simulink model "NB_simulink"  (R2023a)
settings: Solver=VariableStepAuto  StartTime=0.0  StopTime=974  RelTol=1e-3
undefined symbols (not defined in the file): g_i, g_p
libraries: simulink x6
settings Model: Creator=usradmin  LastModifiedBy=usradmin

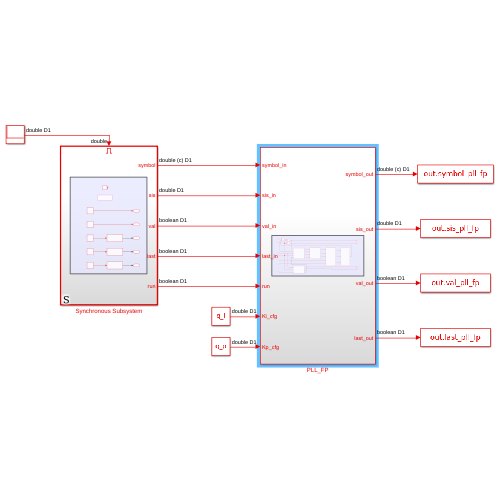
[thumbnail: Simulink's stored preview of the top-level diagram]
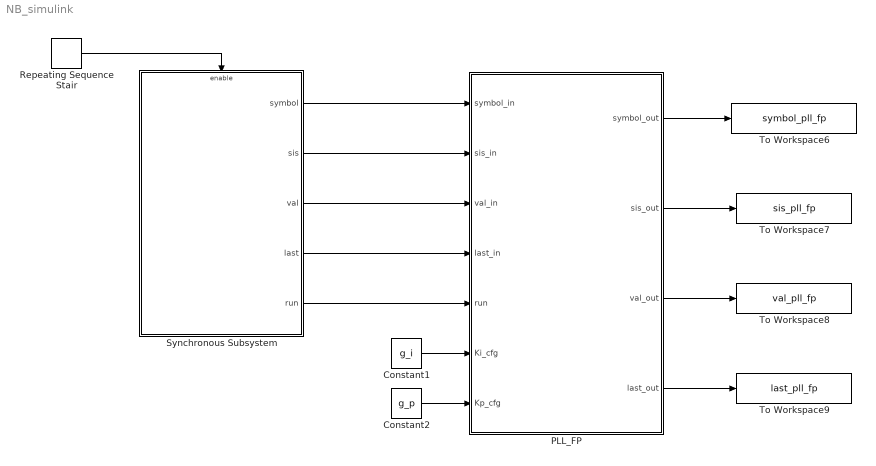
== system NB_simulink ==
  Constant1 : Constant  Value=g_i  SampleTime=-1
  Constant2 : Constant  Value=g_p  SampleTime=-1
  PLL_FP : Subsystem
  Repeating Sequence Stair : simulink/Sources/Repeating Sequence Stair  OutValues=1  tsamp=1  OutMin=[]  OutMax=[]  OutDataTypeStr=double  OutputDataTypeScalingMode=double  OutDataType=fixdt(0,8)  ConRadixGroup=Best Precision: Vector-wise  OutScaling=2^-12
  Synchronous Subsystem : Subsystem
  To Workspace6 : ToWorkspace  VariableName=symbol_pll_fp  SampleTime=-1
      settings: Save2DSignal=2-D array (concatenate along first dimension)
  To Workspace7 : ToWorkspace  VariableName=sis_pll_fp  SampleTime=-1
      settings: Save2DSignal=2-D array (concatenate along first dimension)
  To Workspace8 : ToWorkspace  VariableName=val_pll_fp  SampleTime=-1
      settings: Save2DSignal=2-D array (concatenate along first dimension)
  To Workspace9 : ToWorkspace  VariableName=last_pll_fp  SampleTime=-1
      settings: Save2DSignal=2-D array (concatenate along first dimension)
  wires:
  Repeating Sequence Stair/1 -> Synchronous Subsystem/Enable
  Synchronous Subsystem/1(symbol) -> PLL_FP/1(symbol_in)
  PLL_FP/1(symbol_out) -> To Workspace6/1
  Synchronous Subsystem/4(last) -> PLL_FP/4(last_in)
  PLL_FP/3(val_out) -> To Workspace8/1
  PLL_FP/4(last_out) -> To Workspace9/1
  Constant1/1 -> PLL_FP/6(Ki_cfg)
  Constant2/1 -> PLL_FP/7(Kp_cfg)
  Synchronous Subsystem/2(sis) -> PLL_FP/2(sis_in)
  Synchronous Subsystem/5(run) -> PLL_FP/5(run)
  Synchronous Subsystem/3(val) -> PLL_FP/3(val_in)
  PLL_FP/2(sis_out) -> To Workspace7/1

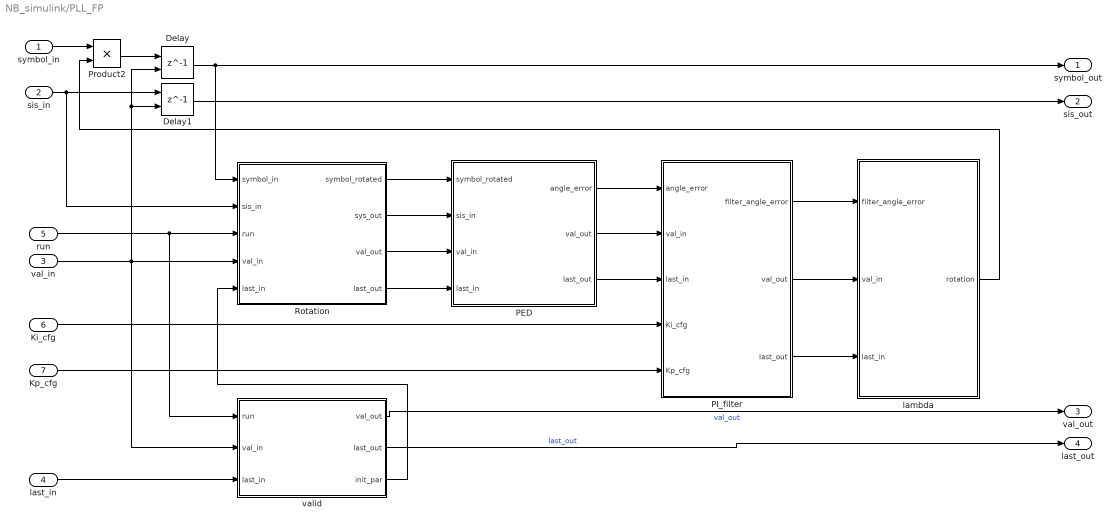
== system NB_simulink/PLL_FP ==
  symbol_in : Inport
  sis_in : Inport  Port=2
  val_in : Inport  Port=3
  last_in : Inport  Port=4
  run : Inport  Port=5
  Ki_cfg : Inport  Port=6
  Kp_cfg : Inport  Port=7
  Delay : Delay  DelayLength=1  InitialCondition=0  ShowEnablePort=on
      settings: InputPortMap=u0,e6
  Delay1 : Delay  DelayLength=1  InitialCondition=0  ShowEnablePort=on
      settings: InputPortMap=u0,e6
  PED : Subsystem
  PI_filter : Subsystem
  Product2 : Product
  Rotation : Subsystem
  lambda : Subsystem
  valid : MATLAB Function  TreatAsAtomicUnit=on
  symbol_out : Outport
  sis_out : Outport  Port=2
  val_out : Outport  Port=3
  last_out : Outport  Port=4
  wires:
  lambda/1(rotation) -> Product2/2
  PED/1(angle_error) -> PI_filter/1(angle_error)
  PI_filter/1(filter_angle_error) -> lambda/1(filter_angle_error)
  Rotation/1(symbol_rotated) -> PED/1(symbol_rotated)
  Product2/1 -> Delay/1
  symbol_in/1 -> Product2/1
  sis_in/1 -> Delay1/1, Rotation/2(sis_in)
  Rotation/2(sys_out) -> PED/2(sis_in)
  val_in/1 -> Delay1/2, Delay/2, valid/2(val_in), Rotation/4(val_in)
  last_in/1 -> valid/3(last_in)
  Rotation/3(val_out) -> PED/3(val_in)
  Rotation/4(last_out) -> PED/4(last_in)
  PED/2(val_out) -> PI_filter/2(val_in)
  PED/3(last_out) -> PI_filter/3(last_in)
  PI_filter/2(val_out) -> lambda/2(val_in)
  PI_filter/3(last_out) -> lambda/3(last_in)
  Delay/1 -> Rotation/1(symbol_in), symbol_out/1
  valid/1(val_out) -> val_out/1  "val_out"
  valid/2(last_out) -> last_out/1  "last_out"
  Ki_cfg/1 -> PI_filter/4(Ki_cfg)
  Kp_cfg/1 -> PI_filter/5(Kp_cfg)
  run/1 -> valid/1(run), Rotation/3(run)
  Delay1/1 -> sis_out/1
  valid/3(init_par) -> Rotation/5(last_in)

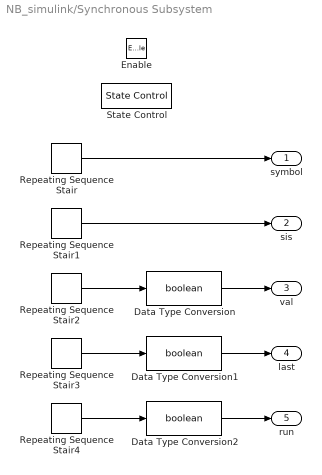
== system NB_simulink/Synchronous Subsystem ==
  Enable : EnablePort  ShowOutputPort=on
  Data Type Conversion : DataTypeConversion  OutDataTypeStr=boolean  SaturateOnIntegerOverflow=off  RndMeth=Floor
  Data Type Conversion1 : DataTypeConversion  OutDataTypeStr=boolean  SaturateOnIntegerOverflow=off  RndMeth=Floor
  Data Type Conversion2 : DataTypeConversion  OutDataTypeStr=boolean  SaturateOnIntegerOverflow=off  RndMeth=Floor
  Repeating Sequence Stair : simulink/Sources/Repeating Sequence Stair  OutValues=symbol_cc  tsamp=1  OutMin=[]  OutMax=[]  OutDataTypeStr=double  OutputDataTypeScalingMode=double  OutDataType=fixdt(0,8)  ConRadixGroup=Best Precision: Vector-wise  OutScaling=2^-12
  Repeating Sequence Stair1 : simulink/Sources/Repeating Sequence Stair  OutValues=sis_cc  tsamp=1  OutMin=[]  OutMax=[]  OutDataTypeStr=double  OutputDataTypeScalingMode=double  OutDataType=fixdt(0,8)  ConRadixGroup=Best Precision: Vector-wise  OutScaling=2^-12
  Repeating Sequence Stair2 : simulink/Sources/Repeating Sequence Stair  OutValues=val_cc  tsamp=1  OutMin=[]  OutMax=[]  OutDataTypeStr=double  OutputDataTypeScalingMode=double  OutDataType=fixdt(0,8)  ConRadixGroup=Best Precision: Vector-wise  OutScaling=2^-12
  Repeating Sequence Stair3 : simulink/Sources/Repeating Sequence Stair  OutValues=last_cc  tsamp=1  OutMin=[]  OutMax=[]  OutDataTypeStr=double  OutputDataTypeScalingMode=double  OutDataType=fixdt(0,8)  ConRadixGroup=Best Precision: Vector-wise  OutScaling=2^-12
  Repeating Sequence Stair4 : simulink/Sources/Repeating Sequence Stair  OutValues=run_cc  tsamp=1  OutMin=[]  OutMax=[]  OutDataTypeStr=double  OutputDataTypeScalingMode=double  OutDataType=fixdt(0,8)  ConRadixGroup=Best Precision: Vector-wise  OutScaling=2^-12
  State Control : StateControl  StateControl=Synchronous
  symbol : Outport  VectorParamsAs1DForOutWhenUnconnected=off
  sis : Outport  Port=2  VectorParamsAs1DForOutWhenUnconnected=off
  val : Outport  Port=3  VectorParamsAs1DForOutWhenUnconnected=off
  last : Outport  Port=4  VectorParamsAs1DForOutWhenUnconnected=off
  run : Outport  Port=5  VectorParamsAs1DForOutWhenUnconnected=off
  wires:
  Repeating Sequence Stair/1 -> symbol/1
  Repeating Sequence Stair1/1 -> sis/1
  Repeating Sequence Stair3/1 -> Data Type Conversion1/1
  Repeating Sequence Stair2/1 -> Data Type Conversion/1
  Repeating Sequence Stair4/1 -> Data Type Conversion2/1
  Data Type Conversion/1 -> val/1
  Data Type Conversion1/1 -> last/1
  Data Type Conversion2/1 -> run/1

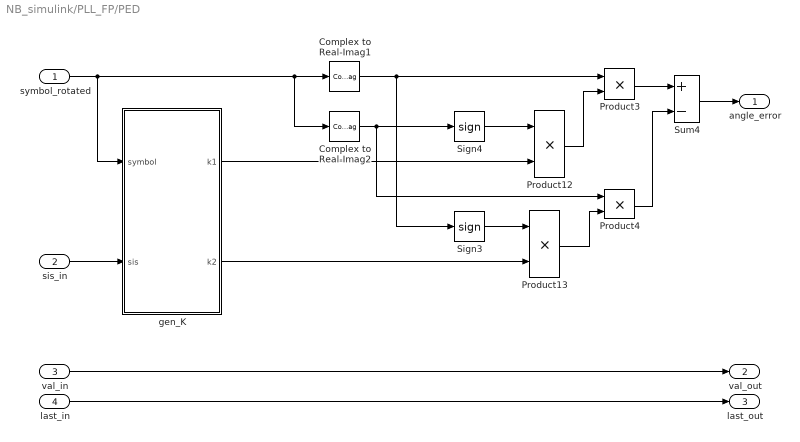
== system NB_simulink/PLL_FP/PED ==
  symbol_rotated : Inport
  sis_in : Inport  Port=2
  val_in : Inport  Port=3
  last_in : Inport  Port=4
  Complex to Real-Imag1 : ComplexToRealImag  Output=Imag
  Complex to Real-Imag2 : ComplexToRealImag  Output=Real
  Product{3..4,12..13} (4 alike) : Product
  Sign3 : Signum
  Sign4 : Signum
  Sum4 : Sum  Inputs=+-
  gen_K : MATLAB Function  TreatAsAtomicUnit=on
  angle_error : Outport
  val_out : Outport  Port=2
  last_out : Outport  Port=3
  wires:
  Product3/1 -> Sum4/1
  Product12/1 -> Product3/2
  gen_K/2(k2) -> Product13/2
  gen_K/1(k1) -> Product12/2
  Sum4/1 -> angle_error/1
  Product4/1 -> Sum4/2
  Sign3/1 -> Product13/1
  Sign4/1 -> Product12/1
  symbol_rotated/1 -> gen_K/1(symbol), Complex to Real-Imag2/1, Complex to Real-Imag1/1
  Complex to Real-Imag1/1 -> Product3/1, Sign3/1
  Complex to Real-Imag2/1 -> Sign4/1, Product4/1
  Product13/1 -> Product4/2
  sis_in/1 -> gen_K/2(sis)
  val_in/1 -> val_out/1
  last_in/1 -> last_out/1

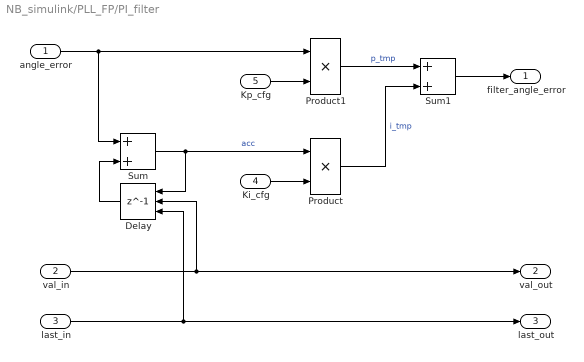
== system NB_simulink/PLL_FP/PI_filter ==
  angle_error : Inport
  val_in : Inport  Port=2
  last_in : Inport  Port=3
  Ki_cfg : Inport  Port=4
  Kp_cfg : Inport  Port=5
  Delay : Delay  DelayLength=1  ExternalReset=Level  ShowEnablePort=on
      settings: InputPortMap=u0,e6,r5
  Product : Product
  Product1 : Product
  Sum : Sum
  Sum1 : Sum
  filter_angle_error : Outport
  val_out : Outport  Port=2
  last_out : Outport  Port=3
  wires:
  Sum/1 -> Delay/1, Product/1  "acc"
  Delay/1 -> Sum/2
  Product1/1 -> Sum1/1  "p_tmp"
  Sum1/1 -> filter_angle_error/1
  angle_error/1 -> Sum/1, Product1/1
  Product/1 -> Sum1/2  "i_tmp"
  val_in/1 -> Delay/2, val_out/1
  last_in/1 -> Delay/3, last_out/1
  Ki_cfg/1 -> Product/2
  Kp_cfg/1 -> Product1/2

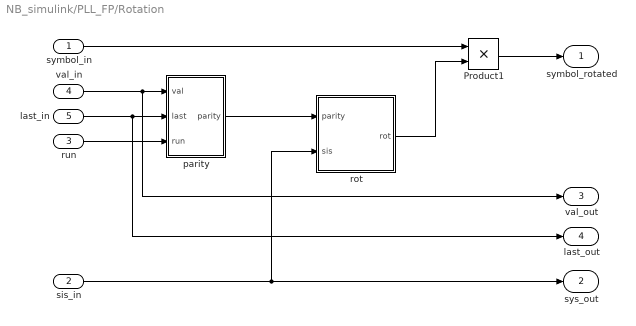
== system NB_simulink/PLL_FP/Rotation ==
  symbol_in : Inport
  sis_in : Inport  Port=2
  run : Inport  Port=3
  val_in : Inport  Port=4
  last_in : Inport  Port=5
  Product1 : Product
  parity : Subsystem
  rot : MATLAB Function  TreatAsAtomicUnit=on
  symbol_rotated : Outport
  sys_out : Outport  Port=2
  val_out : Outport  Port=3
  last_out : Outport  Port=4
  wires:
  Product1/1 -> symbol_rotated/1
  symbol_in/1 -> Product1/1
  sis_in/1 -> rot/2(sis), sys_out/1
  rot/1(rot) -> Product1/2
  val_in/1 -> val_out/1, parity/1(val)
  last_in/1 -> last_out/1, parity/2(last)
  parity/1(parity) -> rot/1(parity)
  run/1 -> parity/3(run)

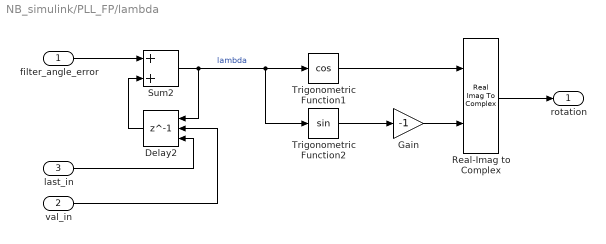
== system NB_simulink/PLL_FP/lambda ==
  filter_angle_error : Inport
  val_in : Inport  Port=2
  last_in : Inport  Port=3
  Delay2 : Delay  DelayLength=1  ExternalReset=Level  ShowEnablePort=on
      settings: InputPortMap=u0,e6,r5
  Gain : Gain  Gain=-1
  Real-Imag to Complex : RealImagToComplex
  Sum2 : Sum
  Trigonometric Function1 : Trigonometry  Operator=cos
  Trigonometric Function2 : Trigonometry
  rotation : Outport
  wires:
  Sum2/1 -> Trigonometric Function1/1, Trigonometric Function2/1, Delay2/1  "lambda"
  Real-Imag to Complex/1 -> rotation/1
  Delay2/1 -> Sum2/2
  filter_angle_error/1 -> Sum2/1
  Trigonometric Function1/1 -> Real-Imag to Complex/1
  Trigonometric Function2/1 -> Gain/1
  Gain/1 -> Real-Imag to Complex/2
  last_in/1 -> Delay2/3
  val_in/1 -> Delay2/2

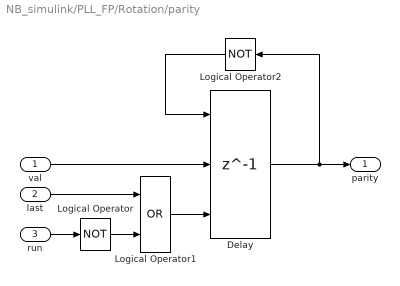
== system NB_simulink/PLL_FP/Rotation/parity ==
  val : Inport
  last : Inport  Port=2
  run : Inport  Port=3
  Delay : Delay  DelayLength=1  InitialCondition=0  ExternalReset=Level  ShowEnablePort=on
      settings: InputPortMap=u0,e6,r5
  Logical Operator : Logic  Operator=NOT  AllPortsSameDT=off  OutDataTypeStr=boolean
  Logical Operator1 : Logic  Operator=OR  AllPortsSameDT=off  OutDataTypeStr=boolean
  Logical Operator2 : Logic  Operator=NOT  AllPortsSameDT=off  OutDataTypeStr=boolean
  parity : Outport
  wires:
  Delay/1 -> Logical Operator2/1, parity/1
  Logical Operator2/1 -> Delay/1
  val/1 -> Delay/2
  last/1 -> Logical Operator1/1
  Logical Operator1/1 -> Delay/3
  run/1 -> Logical Operator/1
  Logical Operator/1 -> Logical Operator1/2

== matlab function NB_simulink/PLL_FP/Rotation/rot ==
  data: parity input; rot output; sis input
function rot = func_rot(parity, sis)
% -------------------------------------------------------------------------
% Function rot
% -------------------------------------------------------------------------
    %#codegen
    if (sis==1)
        if (parity == 0)  % par
            rot = (0 + 1i);
        else              % impar
            rot = (1 + 0i);
        end   
    elseif (sis==2)
        if (parity == 0) % par
            rot = (1 + 0i);
        else             % impar
            rot = (cos(pi/4) + 1i*(sin(pi/4)));
        end  
    else
        if (parity == 0) % par
            rot = (1 + 0i);
        else             % impar
            rot = (cos(pi/8) + 1i*(sin(pi/8)));
        end 
    end 
end
% -------------------------------------------------------------------------

== matlab function NB_simulink/PLL_FP/valid ==
  data: run input; val_in input; last_in input; val_out output; last_out output; init_par output
function [val_out, last_out, init_par] = func_valid(run, val_in, last_in)
% -------------------------------------------------------------------------
% Function valid
% -------------------------------------------------------------------------
    % persistent variable for the state 
    persistent count;
    if isempty(count)
        count = uint16(0);
    end

    % persistent variable for the state 
    persistent count_dwell;
    if isempty(count_dwell)
        count_dwell = uint8(0);
    end

    persistent mask_int;
    if isempty(mask_int)
        mask_int = false;
    end

    persistent init_par_int;
    if isempty(init_par_int)
        init_par_int = false;
    end

    % counting up
    if (not(run))
        count = uint16(0);
    elseif (val_in)
        count = count + uint16(1);
        % limit 
        if (last_in || count > uint16(946))
            count = uint16(0);
        end
    end

    % counting dwell
    if (not(run))
        count_dwell = uint8(0);
    elseif (val_in && count > uint16(946))
        count_dwell = count_dwell + uint8(1);
        % limit to four bits
        if (last_in)
            count_dwell = uint8(0);
        end
    end

    % Calculate the mask
    if (count == uint16(107) || ...
        count == uint16(107+157) || ...
        count == uint16(107+157+11) || ...
        count == uint16(107+157+11+157) || ...
        count == uint16(107+157+11+157+11) || ...
        count == uint16(107+157+11+157+11+157) || ...
        count == uint16(107+157+11+157+11+157+11) || ...
        count == uint16(107+157+11+157+11+157+11+157) || ...
        count == uint16(107+157+11+157+11+157+11+157+11) || ...
        count == uint16(107+157+11+157+11+157+11+157+11+157))
        mask_int = not(mask_int);
    end

    % calculate last
    if (count_dwell == uint8(4) && count == uint16(935))
        last_out = true;
    else
        last_out = false;
    end

    % calculate last
    if (count == uint16(946) && val_in)
        init_par_int = true;
    else
        init_par_int = false;
    end

    val_out = mask_int && val_in;
    init_par = init_par_int || val_in;
end 
% -------------------------------------------------------------------------

== matlab function NB_simulink/PLL_FP/PED/gen_K ==
  data: symbol input; k1 output; sis input; k2 output
function [k1, k2] = func_gen_K(symbol, sis)
% -------------------------------------------------------------------------
% Function gen_K
% -------------------------------------------------------------------------
    real_tmp = abs(real(symbol));
    imag_tmp = abs(imag(symbol));
    
    % Determina quien es mayor la parte real o imaginaria
    if (real_tmp < imag_tmp)
        tmp = 1;
    else
        tmp = 0;
    end
    
    % calcula k1 y k2 
    if (sis == 1)
       k1 = 1;
       k2 = 0;
    elseif (sis == 2)
       k1 = 1;
       k2 = 1;
    elseif (sis == 3 && tmp == 1)
       k1 = sqrt(2)-1;
       k2 = 1;
    else
       k1 = 1;
       k2 = sqrt(2)-1;
    end
end
% -------------------------------------------------------------------------
